simulink model "lateral_model_traj_control"  (R2020a)
settings: Solver=ode45  StartTime=0.0  StopTime=Tfinal  RelTol=1e-3  EnableMultiTasking=on
undefined symbols (not defined in the file or in its folder): Calpha, Izz, K, lf, lr, m, mu, Tc, Vy0, X0, Y0, Yaw0, yaw_rate0
settings Model: Creator=user  LastModifiedBy=USER
settings SolverCC: ZeroCrossAlgorithm=Non-adaptive
settings DataIOCC: LimitDataPoints=on  SaveFormat=Array  SignalLoggingSaveFormat=ModelDataLogs  ReturnWorkspaceOutputs=off
settings OptimizationCC: ExpressionDepthLimit=2147483647  InitFltsAndDblsToZero=on  LifeSpan=inf
settings DebuggingCC: UnderspecifiedInitializationDetection=Classic  MergeDetectMultiDrivingBlocksExec=none  SolverPrmCheckMsg=warning  FcnCallInpInsideContextMsg=warning  StateNameClashWarn=warning  SFUnexpectedBacktrackingDiag=warning  SFNoUnconditionalDefaultTransitionDiag=warning  SFExecutionAtInitializationDiag=none  ArithmeticOperatorsInVariantConditions=warning
settings HardwareCC: ProdBitPerPointer=32  ProdBitPerSizeT=32  ProdBitPerPtrDiffT=32  ProdLargestAtomicFloat=None  ProdIntDivRoundTo=Undefined  ProdEndianess=Unspecified  ProdWordSize=32  ProdHWDeviceType=32-bit Generic
settings ModelReferenceCC: PropagateSignalLabelsOutOfModel=off
settings SFSimCC: CustomCodeUndefinedFunction=UseInterfaceOnly
settings CodeAppCC: StateflowObjectComments=on
settings GRTTargetCC: TargetLangStandard=C89/C90 (ANSI)  CombineOutputUpdateFcns=off  GRTInterface=on
settings ConfigComp: CovMetricSettings=dw  CovHtmlReporting=on  CovSaveCumulativeToWorkspaceVar=on  CovSaveSingleToWorkspaceVar=on

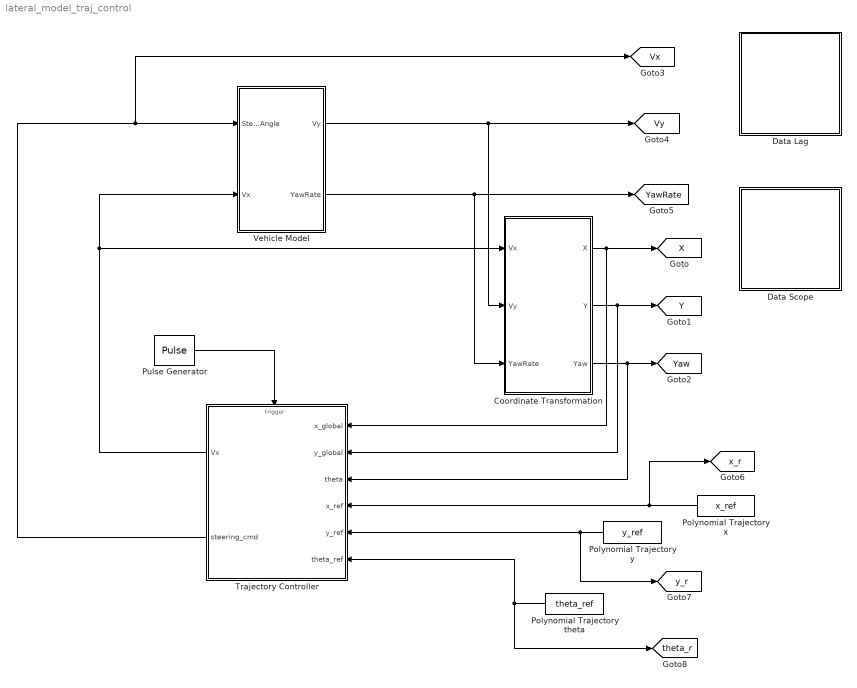
== system lateral_model_traj_control ==
  Coordinate Transformation : Subsystem
  Data Lag : Subsystem
  Data Scope : Subsystem
  Polynomial Trajectory theta : FromWorkspace  VariableName=theta_ref
  Polynomial Trajectory x : FromWorkspace  VariableName=x_ref
  Polynomial Trajectory y : FromWorkspace  VariableName=y_ref
  Pulse Generator : DiscretePulseGenerator  PulseType=Time based  Period=Tc  PulseWidth=50
  Trajectory Controller : Subsystem
  Vehicle Model : Subsystem
  tag scope: Vx=global, Vy=global, X=global, Y=global, Yaw=global, YawRate=global, theta_r=global, x_r=global, y_r=global
  wires:
  Vehicle Model/1(Vy) -> Coordinate Transformation/2(Vy), [Vy]
  Vehicle Model/2(YawRate) -> Coordinate Transformation/3(YawRate), [YawRate]
  Coordinate Transformation/1(X) -> Trajectory Controller/1(x_global), [X]
  Coordinate Transformation/2(Y) -> Trajectory Controller/2(y_global), [Y]
  Coordinate Transformation/3(Yaw) -> Trajectory Controller/3(theta), [Yaw]
  Pulse Generator/1 -> Trajectory Controller/Trigger
  Trajectory Controller/1(Vx) -> Coordinate Transformation/1(Vx), Vehicle Model/2(Vx)
  Trajectory Controller/2(steering_cmd) -> [Vx], Vehicle Model/1(Steering_Angle)
  Polynomial Trajectory theta/1 -> Trajectory Controller/6(theta_ref), [theta_r]
  Polynomial Trajectory x/1 -> [x_r], Trajectory Controller/4(x_ref)
  Polynomial Trajectory y/1 -> [y_r], Trajectory Controller/5(y_ref)

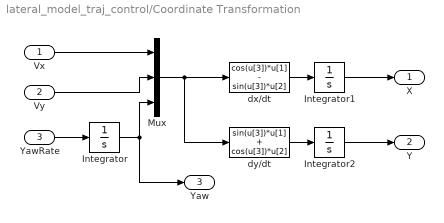
== system lateral_model_traj_control/Coordinate Transformation ==
  Vx : Inport
  Vy : Inport  Port=2
  YawRate : Inport  Port=3
  Integrator : Integrator  InitialCondition=Yaw0
  Integrator1 : Integrator  InitialCondition=X0
  Integrator2 : Integrator  InitialCondition=Y0
  Mux : Mux  Inputs=3
  dx/dt : Fcn  Expr=cos(u[3])*u[1] - sin(u[3])*u[2]
  dy/dt : Fcn  Expr=sin(u[3])*u[1] + cos(u[3])*u[2]
  X : Outport  VectorParamsAs1DForOutWhenUnconnected=off
  Y : Outport  Port=2  VectorParamsAs1DForOutWhenUnconnected=off
  Yaw : Outport  Port=3  VectorParamsAs1DForOutWhenUnconnected=off
  wires:
  YawRate/1 -> Integrator/1
  Vx/1 -> Mux/1
  Vy/1 -> Mux/2
  Integrator/1 -> Mux/3, Yaw/1
  Mux/1 -> dx/dt/1, dy/dt/1
  dx/dt/1 -> Integrator1/1
  Integrator1/1 -> X/1
  dy/dt/1 -> Integrator2/1
  Integrator2/1 -> Y/1

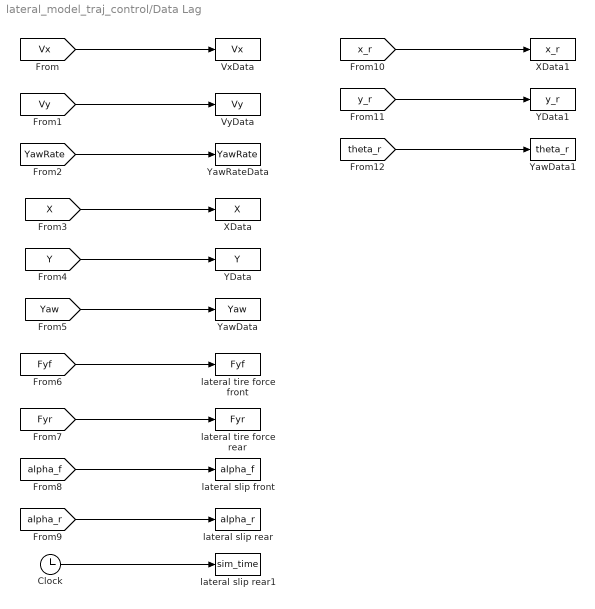
== system lateral_model_traj_control/Data Lag ==
  Clock : Clock
  VxData : ToWorkspace  VariableName=Vx  SampleTime=-1
  VyData : ToWorkspace  VariableName=Vy  SampleTime=-1
  XData : ToWorkspace  VariableName=X  SampleTime=-1
  XData1 : ToWorkspace  VariableName=x_r  SampleTime=-1
  YData : ToWorkspace  VariableName=Y  SampleTime=-1
  YData1 : ToWorkspace  VariableName=y_r  SampleTime=-1
  YawData : ToWorkspace  VariableName=Yaw  SampleTime=-1
  YawData1 : ToWorkspace  VariableName=theta_r  SampleTime=-1
  YawRateData : ToWorkspace  VariableName=YawRate  SampleTime=-1
  lateral slip front : ToWorkspace  VariableName=alpha_f  SampleTime=-1
  lateral slip rear : ToWorkspace  VariableName=alpha_r  SampleTime=-1
  lateral slip rear1 : ToWorkspace  VariableName=sim_time  SampleTime=-1
  lateral tire force front : ToWorkspace  VariableName=Fyf  SampleTime=-1
  lateral tire force rear : ToWorkspace  VariableName=Fyr  SampleTime=-1
  wires:
  [Vx] -> VxData/1
  [Vy] -> VyData/1
  [YawRate] -> YawRateData/1
  [X] -> XData/1
  [Y] -> YData/1
  [Yaw] -> YawData/1
  [Fyf] -> lateral tire force front/1
  [Fyr] -> lateral tire force rear/1
  [alpha_f] -> lateral slip front/1
  [alpha_r] -> lateral slip rear/1
  Clock/1 -> lateral slip rear1/1
  [x_r] -> XData1/1
  [y_r] -> YData1/1
  [theta_r] -> YawData1/1

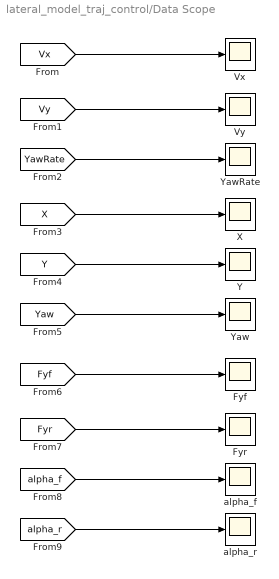
== system lateral_model_traj_control/Data Scope ==
  Fyf : Scope
  Fyr : Scope
  Vx : Scope
  Vy : Scope
  X : Scope
  Y : Scope
  Yaw : Scope
  YawRate : Scope
  alpha_f : Scope
  alpha_r : Scope
  wires:
  [Vx] -> Vx/1
  [Vy] -> Vy/1
  [YawRate] -> YawRate/1
  [X] -> X/1
  [Y] -> Y/1
  [Yaw] -> Yaw/1
  [Fyf] -> Fyf/1
  [Fyr] -> Fyr/1
  [alpha_f] -> alpha_f/1
  [alpha_r] -> alpha_r/1

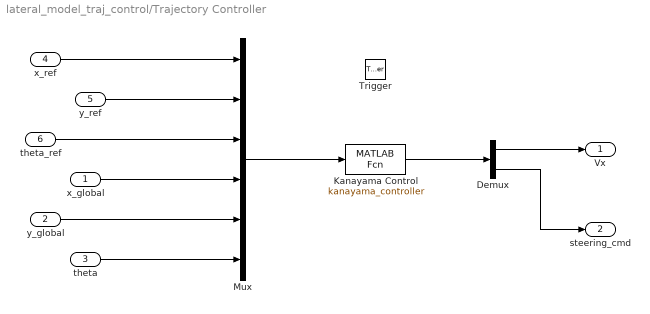
== system lateral_model_traj_control/Trajectory Controller ==
  x_global : Inport
  y_global : Inport  Port=2
  theta : Inport  Port=3
  x_ref : Inport  Port=4
  y_ref : Inport  Port=5
  theta_ref : Inport  Port=6
  Trigger : TriggerPort  VariantControl=(inherit)
  Demux : Demux  Outputs=2
  Kanayama Control : MATLABFcn  MATLABFcn=kanayama_controller
  Mux : Mux  Inputs=6
  Vx : Outport  VectorParamsAs1DForOutWhenUnconnected=off
  steering_cmd : Outport  Port=2  VectorParamsAs1DForOutWhenUnconnected=off
  wires:
  x_ref/1 -> Mux/1
  y_ref/1 -> Mux/2
  theta_ref/1 -> Mux/3
  x_global/1 -> Mux/4
  y_global/1 -> Mux/5
  theta/1 -> Mux/6
  Mux/1 -> Kanayama Control/1
  Kanayama Control/1 -> Demux/1
  Demux/1 -> Vx/1
  Demux/2 -> steering_cmd/1

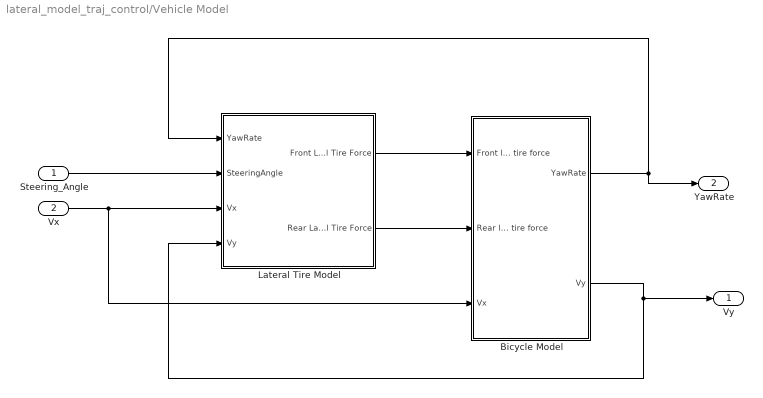
== system lateral_model_traj_control/Vehicle Model ==
  Steering_Angle : Inport
  Vx : Inport  Port=2
  Bicycle Model : Subsystem
  Lateral Tire Model : Subsystem
  Vy : Outport  VectorParamsAs1DForOutWhenUnconnected=off
  YawRate : Outport  Port=2  VectorParamsAs1DForOutWhenUnconnected=off
  wires:
  Steering_Angle/1 -> Lateral Tire Model/2(SteeringAngle)
  Lateral Tire Model/1(Front Lateral Tire Force) -> Bicycle Model/1(Front lateral tire force)
  Lateral Tire Model/2(Rear Lateral Tire Force) -> Bicycle Model/2(Rear lateral tire force)
  Bicycle Model/1(YawRate) -> YawRate/1, Lateral Tire Model/1(YawRate)
  Bicycle Model/2(Vy) -> Vy/1, Lateral Tire Model/4(Vy)
  Vx/1 -> Lateral Tire Model/3(Vx), Bicycle Model/3(Vx)

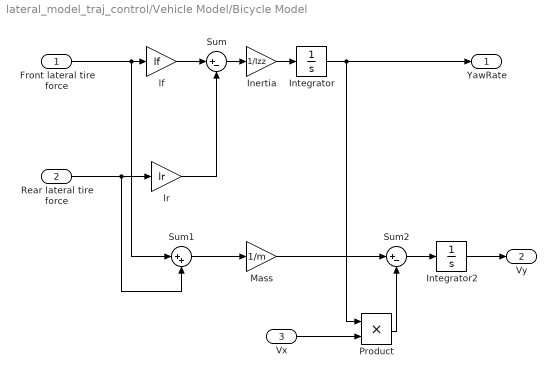
== system lateral_model_traj_control/Vehicle Model/Bicycle Model ==
  Front lateral tire force : Inport
  Rear lateral tire force : Inport  Port=2
  Vx : Inport  Port=3
  Inertia : Gain  Gain=1/Izz
  Integrator : Integrator  InitialCondition=yaw_rate0
  Integrator2 : Integrator  InitialCondition=Vy0
  Mass : Gain  Gain=1/m
  Product : Product  RndMeth=Zero
  Sum : Sum  Inputs=|+-
  Sum1 : Sum  Inputs=|++
  Sum2 : Sum  Inputs=|+-
  lf : Gain  Gain=lf
  lr : Gain  Gain=lr
  YawRate : Outport  VectorParamsAs1DForOutWhenUnconnected=off
  Vy : Outport  Port=2  VectorParamsAs1DForOutWhenUnconnected=off
  wires:
  Front lateral tire force/1 -> lf/1, Sum1/1
  Rear lateral tire force/1 -> lr/1, Sum1/2
  Sum/1 -> Inertia/1
  Inertia/1 -> Integrator/1
  Integrator/1 -> YawRate/1, Product/1
  Sum1/1 -> Mass/1
  Mass/1 -> Sum2/1
  Vx/1 -> Product/2
  Product/1 -> Sum2/2
  Sum2/1 -> Integrator2/1
  Integrator2/1 -> Vy/1
  lf/1 -> Sum/1
  lr/1 -> Sum/2

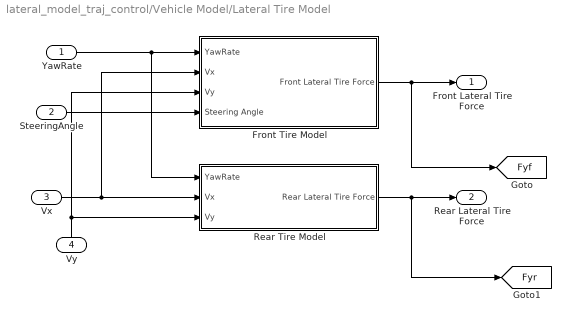
== system lateral_model_traj_control/Vehicle Model/Lateral Tire Model ==
  YawRate : Inport
  SteeringAngle : Inport  Port=2
  Vx : Inport  Port=3
  Vy : Inport  Port=4
  Front Tire Model : Subsystem
  Rear Tire Model : Subsystem
  Front Lateral Tire Force : Outport  VectorParamsAs1DForOutWhenUnconnected=off
  Rear Lateral Tire Force : Outport  Port=2  VectorParamsAs1DForOutWhenUnconnected=off
  tag scope: Fyf=global, Fyr=global
  wires:
  Vx/1 -> Rear Tire Model/2(Vx), Front Tire Model/2(Vx)
  Vy/1 -> Rear Tire Model/3(Vy), Front Tire Model/3(Vy)
  YawRate/1 -> Front Tire Model/1(YawRate), Rear Tire Model/1(YawRate)
  Front Tire Model/1(Front Lateral Tire Force) -> Front Lateral Tire Force/1, [Fyf]
  SteeringAngle/1 -> Front Tire Model/4(Steering Angle)
  Rear Tire Model/1(Rear Lateral Tire Force) -> Rear Lateral Tire Force/1, [Fyr]

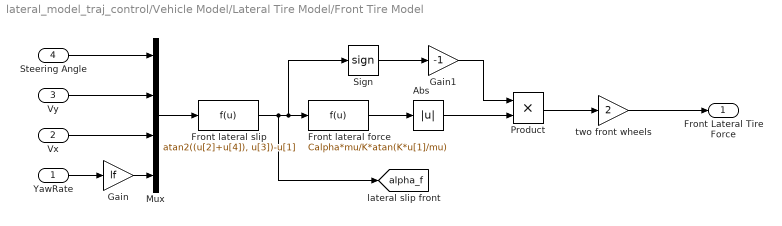
== system lateral_model_traj_control/Vehicle Model/Lateral Tire Model/Front Tire Model ==
  YawRate : Inport
  Vx : Inport  Port=2
  Vy : Inport  Port=3
  Steering Angle : Inport  Port=4
  Abs : Abs
  Front lateral force : Fcn  Expr=Calpha*mu/K*atan(K*u[1]/mu)
  Front lateral slip : Fcn  Expr=atan2((u[2]+u[4]), u[3])-u[1]
  Gain : Gain  Gain=lf
  Gain1 : Gain  Gain=-1
  Mux : Mux
  Product : Product  RndMeth=Zero
  Sign : Signum
  two front wheels : Gain  Gain=2
  Front Lateral Tire Force : Outport  VectorParamsAs1DForOutWhenUnconnected=off
  tag scope: alpha_f=global
  wires:
  Steering Angle/1 -> Mux/1
  Vy/1 -> Mux/2
  Vx/1 -> Mux/3
  YawRate/1 -> Gain/1
  Mux/1 -> Front lateral slip/1
  Gain/1 -> Mux/4
  Front lateral slip/1 -> [alpha_f], Front lateral force/1, Sign/1
  Front lateral force/1 -> Abs/1
  Sign/1 -> Gain1/1
  Gain1/1 -> Product/1
  Abs/1 -> Product/2
  Product/1 -> two front wheels/1
  two front wheels/1 -> Front Lateral Tire Force/1

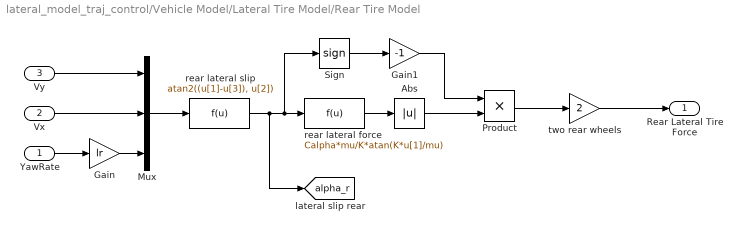
== system lateral_model_traj_control/Vehicle Model/Lateral Tire Model/Rear Tire Model ==
  YawRate : Inport
  Vx : Inport  Port=2
  Vy : Inport  Port=3
  Abs : Abs
  Gain : Gain  Gain=lr
  Gain1 : Gain  Gain=-1
  Mux : Mux  Inputs=3
  Product : Product  RndMeth=Zero
  Sign : Signum
  rear lateral force : Fcn  Expr=Calpha*mu/K*atan(K*u[1]/mu)
  rear lateral slip : Fcn  Expr=atan2((u[1]-u[3]), u[2])
  two rear wheels : Gain  Gain=2
  Rear Lateral Tire Force : Outport  VectorParamsAs1DForOutWhenUnconnected=off
  tag scope: alpha_r=global
  wires:
  rear lateral slip/1 -> [alpha_r], rear lateral force/1, Sign/1
  Gain/1 -> Mux/3
  Mux/1 -> rear lateral slip/1
  YawRate/1 -> Gain/1
  Vy/1 -> Mux/1
  Vx/1 -> Mux/2
  Sign/1 -> Gain1/1
  rear lateral force/1 -> Abs/1
  Gain1/1 -> Product/1
  Abs/1 -> Product/2
  Product/1 -> two rear wheels/1
  two rear wheels/1 -> Rear Lateral Tire Force/1
